simulink model "Simulation_2018"  (R2022b)
settings: Solver=FixedStepAuto  StartTime=0.0  StopTime=Tsim  FixedStep=param.tSample  RelTol=1e-3  EnableMultiTasking=on
StopFcn:
  | run animation
  | run plotSol
values from neighbouring files (symbols this model uses):
  grampc = grampc_update_struct_grampc(grampc,user)    [initData.m]
  param = load_parameter(param)    [script_Simulation.m]
undefined symbols (not defined in the file or in its folder): cost
settings Model: Creator=kaepernick  LastModifiedBy=Khaled
settings SolverCC: AlgebraicLoopSolver=TrustRegion
settings DataIOCC: LimitDataPoints=on  SaveFormat=Array  ReturnWorkspaceOutputs=off
settings OptimizationCC: ExpressionDepthLimit=2147483647  LifeSpan=inf
settings DebuggingCC: UnderspecifiedInitializationDetection=Classic  MergeDetectMultiDrivingBlocksExec=none  SolverPrmCheckMsg=warning  UnconnectedInputMsg=warning  UnconnectedOutputMsg=warning  UnconnectedLineMsg=warning  StateNameClashWarn=warning  SFUnexpectedBacktrackingDiag=warning  SFNoUnconditionalDefaultTransitionDiag=warning  SFExecutionAtInitializationDiag=none  SFMachineParentedDataDiag=warning  ArithmeticOperatorsInVariantConditions=warning
settings HardwareCC: ProdBitPerPointer=32  ProdBitPerSizeT=32  ProdBitPerPtrDiffT=32  ProdLargestAtomicFloat=None  ProdIntDivRoundTo=Undefined  ProdEndianess=Unspecified  ProdWordSize=32  ProdHWDeviceType=32-bit Generic
settings ModelReferenceCC: EnableRefExpFcnMdlSchedulingChecks=on  PropagateSignalLabelsOutOfModel=off
settings SFSimCC: SimUseLocalCustomCode=off  CustomCodeUndefinedFunction=UseInterfaceOnly
settings RTWCC: RTWUseLocalCustomCode=off
settings CodeAppCC: StateflowObjectComments=on
settings GRTTargetCC: TargetLangStandard=C89/C90 (ANSI)
settings ConfigComp: CovMetricSettings=dw  CovSaveCumulativeToWorkspaceVar=on  CovSaveSingleToWorkspaceVar=on  CovExternalEMLEnable=off

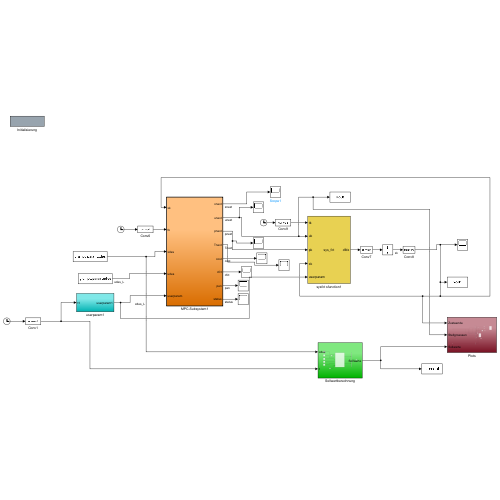
[thumbnail: Simulink's stored preview of the top-level diagram]
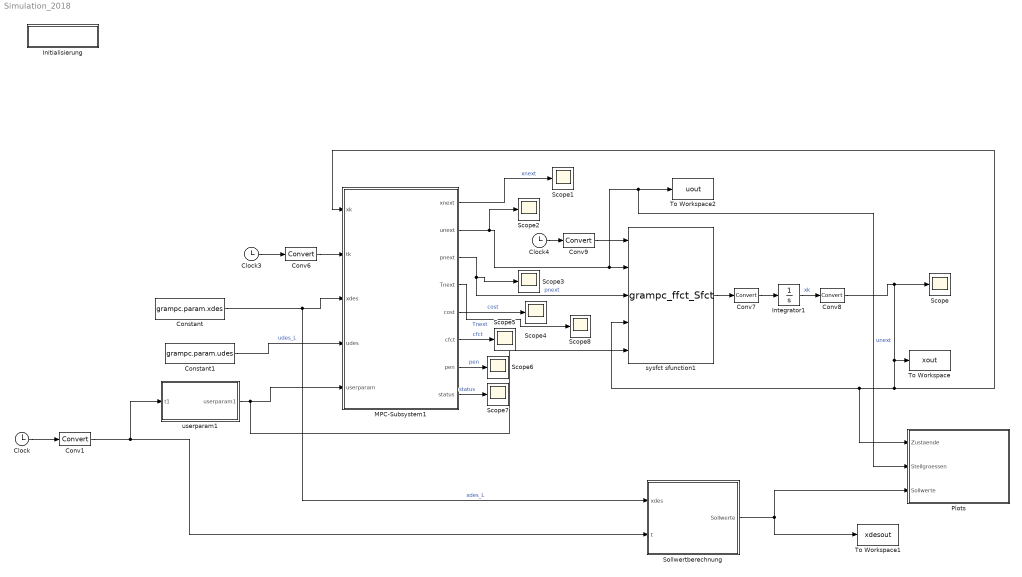
== system Simulation_2018 ==
  Clock : Clock
  Clock3 : Clock
  Clock4 : Clock
  Constant : Constant  Value=grampc.param.xdes
  Constant1 : Constant  Value=grampc.param.udes
  Conv{1,6..9} (5 alike) : DataTypeConversion  SaturateOnIntegerOverflow=off  RndMeth=Floor
  Initialisierung : Subsystem
      settings: OpenFcn=run script_Simulation
  Integrator1 : Integrator  InitialCondition=double(grampc.param.x0)
  MPC-Subsystem1 : Subsystem  TreatAsAtomicUnit=on  SystemSampleTime=double(grampc.param.dt)
  Plots : Subsystem
  Scope{,1..8} (9 alike) : Scope
  Sollwertberechnung : Subsystem
  To Workspace : ToWorkspace  VariableName=xout  SaveFormat=Timeseries  SampleTime=-1
  To Workspace1 : ToWorkspace  VariableName=xdesout  SaveFormat=Timeseries  SampleTime=-1
  To Workspace2 : ToWorkspace  VariableName=uout  SaveFormat=Timeseries  SampleTime=-1
  sysfct sfunction1 : S-Function  FunctionName=grampc_ffct_Sfct  SFunctionDeploymentMode=off  EnableBusSupport=off
      mask Display:
      | port_label('input',1,'tk')
      | port_label('input',2,'uk')
      | port_label('input',3,'pk')
      | port_label('input',4,'xk')
      | port_label('input',5,'userparam')
      | 
      | port_label('output',1,'dfdx')
      | 
      | 
      | disp('sys_fct')
  userparam1 : Subsystem
  wires:
  Sollwertberechnung/1(Sollwerte) -> To Workspace1/1, Plots/3(Sollwerte)
  Clock/1 -> Conv1/1
  Conv1/1 -> userparam1/1(t1), Sollwertberechnung/2(t)
  Constant/1 -> MPC-Subsystem1/3(xdes), Sollwertberechnung/1(xdes)  "xdes_L"
  Conv6/1 -> MPC-Subsystem1/2(tk)
  Clock3/1 -> Conv6/1
  Constant1/1 -> MPC-Subsystem1/4(udes)  "udes_L"
  userparam1/1(userparam1) -> sysfct sfunction1/5, MPC-Subsystem1/5(userparam)
  sysfct sfunction1/1 -> Conv7/1
  Integrator1/1 -> Conv8/1  "xk"
  Conv7/1 -> Integrator1/1
  Clock4/1 -> Conv9/1
  Conv9/1 -> sysfct sfunction1/1
  MPC-Subsystem1/2(unext) -> Scope2/1, Plots/2(Stellgroessen), To Workspace2/1, sysfct sfunction1/2  "unext"
  MPC-Subsystem1/3(pnext) -> Scope3/1, sysfct sfunction1/3  "pnext"
  Conv8/1 -> To Workspace/1, Plots/1(Zustaende), sysfct sfunction1/4, MPC-Subsystem1/1(xk), Scope/1
  MPC-Subsystem1/1(xnext) -> Scope1/1  "xnext"
  MPC-Subsystem1/5(cost) -> Scope4/1  "cost"
  MPC-Subsystem1/6(cfct) -> Scope5/1  "cfct"
  MPC-Subsystem1/7(pen) -> Scope6/1  "pen"
  MPC-Subsystem1/8(status) -> Scope7/1  "status"
  MPC-Subsystem1/4(Tnext) -> Scope8/1  "Tnext"

== system Simulation_2018/Initialisierung ==

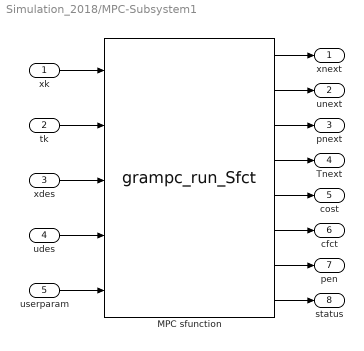
== system Simulation_2018/MPC-Subsystem1 ==
  xk : Inport
  tk : Inport  Port=2
  xdes : Inport  Port=3
  udes : Inport  Port=4
  userparam : Inport  Port=5
  MPC sfunction : S-Function  FunctionName=grampc_run_Sfct  Parameters=grampc_sdata.intoptidx grampc_sdata.intopt grampc_sdata.numoptidx grampc_sdata.numopt grampc_sdata.numparamidx grampc_sdata.numparam  SFunctionDeploymentMode=off  EnableBusSupport=off
      mask Display:
      | port_label('input',1,'x0')
      | port_label('input',2,'t0')
      | port_label('input',3,'xdes')
      | port_label('input',4,'udes')
      | port_label('input',5,'userparam')
      | 
      | port_label('output',1,'xnext')
      | port_label('output',2,'unext')
      | port_label('output',3,'pnext')
      | port_label('output',4,'Tnext')
      | port_label('output',5,'cost')
      | port_label('output',6,'||cfct||')
      | port_label('output',7,'||pen||')
      | port_label('output',8,'status')
      | 
      | disp('GRAMPC')
  xnext : Outport  VectorParamsAs1DForOutWhenUnconnected=off
  unext : Outport  Port=2  VectorParamsAs1DForOutWhenUnconnected=off
  pnext : Outport  Port=3  VectorParamsAs1DForOutWhenUnconnected=off
  Tnext : Outport  Port=4  VectorParamsAs1DForOutWhenUnconnected=off
  cost : Outport  Port=5  VectorParamsAs1DForOutWhenUnconnected=off
  cfct : Outport  Port=6  VectorParamsAs1DForOutWhenUnconnected=off
  pen : Outport  Port=7  VectorParamsAs1DForOutWhenUnconnected=off
  status : Outport  Port=8  VectorParamsAs1DForOutWhenUnconnected=off
  wires:
  xk/1 -> MPC sfunction/1
  MPC sfunction/1 -> xnext/1
  MPC sfunction/8 -> status/1
  MPC sfunction/7 -> pen/1
  xdes/1 -> MPC sfunction/3
  MPC sfunction/6 -> cfct/1
  udes/1 -> MPC sfunction/4
  MPC sfunction/5 -> cost/1
  MPC sfunction/3 -> pnext/1
  MPC sfunction/4 -> Tnext/1
  MPC sfunction/2 -> unext/1
  tk/1 -> MPC sfunction/2
  userparam/1 -> MPC sfunction/5

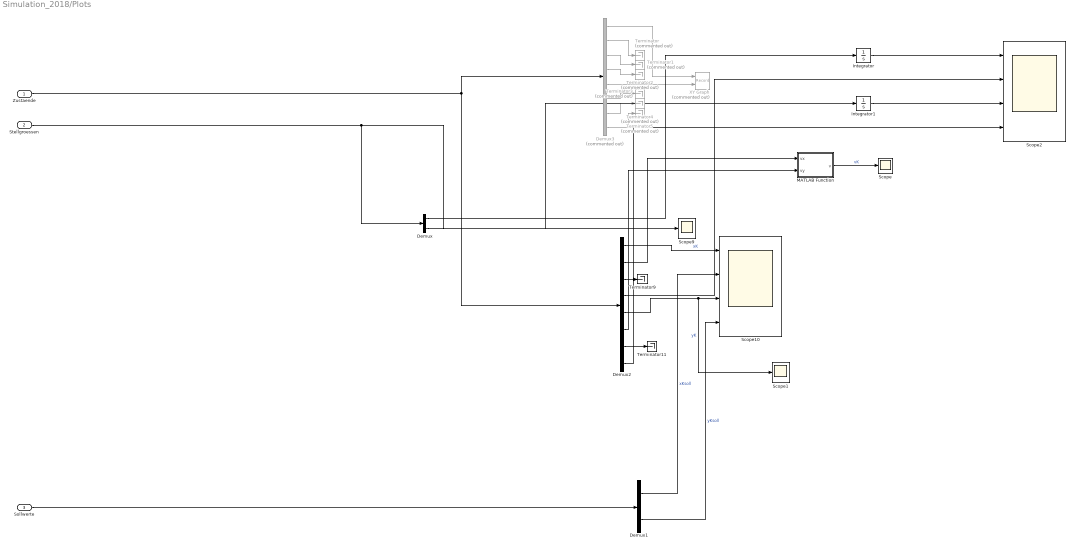
== system Simulation_2018/Plots ==
  Zustaende : Inport
  Stellgroessen : Inport  Port=2
  Sollwerte : Inport  Port=3
  Demux : Demux  Outputs=2
  Demux1 : Demux  Outputs=2
  Demux2 : Demux  Outputs=8
  Demux3 : Demux  Commented=on  Outputs=8
  Integrator : Integrator
  Integrator1 : Integrator
  MATLAB Function : MATLAB Function  TreatAsAtomicUnit=on
  Scope : Scope
  Scope1 : Scope
  Scope10 : Scope  NumInputPorts=4
  Scope2 : Scope  NumInputPorts=4
  Scope9 : Scope
  Terminator{,1..5} (6 alike) : Terminator  Commented=on
  Terminator11 : Terminator
  Terminator9 : Terminator
  XY Graph : Record  Commented=on  FileSettingsInternal="{\"entries\":[{\"content\":{\"excelSettings\":{\"content\":{},\"type\":\"Streamout.ExcelSettings\"}},\"type\":\"Streamout.FileSettingStorage\",\"uuid\":\"823fc073-f533-4fd2-9304-fd0138ba539a\"}],\"packageUris\":[\"http://schema.mathworks.com/mf0/streamout_blocks/R2020a\"],\"version\":\"1.0\"}"  Layout=[1 1]  SignalsInternal="{\"entries\":[{\"content\":{\"signals\":[{\"content\":{\"blockPath\":[\"Simulation_2018/Plots/XY Graph\"],\"channel\":[],\"dimensions\":[1],\"domain\":\"Simulation_2018/Plots/XY Graph\",\"lineColor\":\"#a2142f\",\"plots\":[1],\"port\":1,\"sid\":[],\"signalID\":122,\"signalName\":\"XY Graph:1\"},\"type\":\"RecordBlkView.Signal\",\"uuid\":\"b63b5092-08b6-42c8-9337-63953eef31e7\"},{\"content\":{\"blockPath\":[\"Simulation_2018/Plots/XY Graph\"],\"channel\":[],\"dimensions\":[1],\"domain\":\"Simulation_2018/Plots/XY Graph\",\"lineColor\":\"#139fff\",\"plots\":[1],\"port\":2,\"sid\":[],\"signalID\":125,\"signalName\":\"XY Graph:2\"},\"type\":\"RecordBlkView.Signal\",\"uuid\":\"3b01fe3b-a78f-42cf-b061-e2f77cf29949\"}]},\"type\":\"RecordBlkView.InputSignals\",\"uuid\":\"8815cdad-7d21-4a19-9d66-34a392429214\"}],\"packageUris\":[\"http://schema.mathworks.com/mf0/streamout_blocks/R2020a\"],\"version\":\"1.0\"}"  VisualizationBindings="{\"xyplotplugin\":{\"info\":[{\"series\":[{\"bindingParametersList\":[{\"parameter\":\"X-Axis\",\"signalID\":122,\"signalName\":\"XY Graph:1\"},{\"parameter\":\"Y-Axis\",\"signalID\":125,\"signalName\":\"XY Graph:2\"}],\"seriesID\":53896}],\"subplotID\":1}]}}"  CompatibilityTag=XY  st=-1
  wires:
  Demux2/6 -> MATLAB Function/2(vy)
  Demux1/2 -> Scope10/4  "yKsoll"
  Demux2/5 -> Scope1/1, Scope10/3  "yK"
  Demux2/2 -> MATLAB Function/1(vx)
  Demux3/1 -> XY Graph/1
  Demux2/1 -> Scope10/1  "xK"
  Demux3/5 -> XY Graph/2
  Demux1/1 -> Scope10/2  "xKsoll"
  Zustaende/1 -> Demux2/1, Demux3/1
  Sollwerte/1 -> Demux1/1
  Stellgroessen/1 -> Demux/1, Scope9/1
  Demux3/2 -> Terminator/1
  Demux3/3 -> Terminator1/1
  Demux3/4 -> Terminator2/1
  Demux3/6 -> Terminator3/1
  Demux3/7 -> Terminator4/1
  Demux3/8 -> Terminator5/1
  Demux2/3 -> Terminator9/1
  Demux2/4 -> Scope2/2
  Demux2/7 -> Terminator11/1
  Demux2/8 -> Scope2/4
  Demux/1 -> Integrator/1
  Demux/2 -> Integrator1/1
  Integrator/1 -> Scope2/1
  Integrator1/1 -> Scope2/3
  MATLAB Function/1(v) -> Scope/1  "vK"

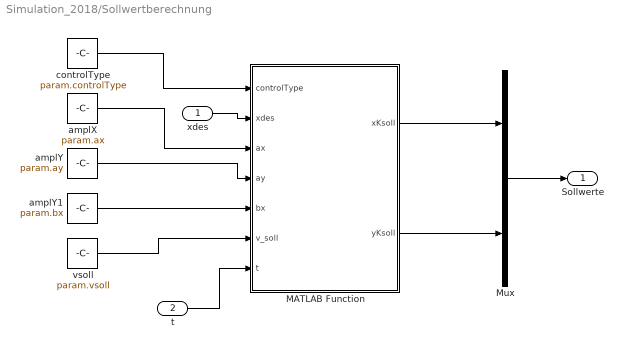
== system Simulation_2018/Sollwertberechnung ==
  xdes : Inport
  t : Inport  Port=2
  MATLAB Function : MATLAB Function  TreatAsAtomicUnit=on
  Mux : Mux  Inputs=2
  amplX : Constant  Value=param.ax
  amplY : Constant  Value=param.ay
  amplY1 : Constant  Value=param.bx
  controlType : Constant  Value=param.controlType
  vsoll : Constant  Value=param.vsoll
  Sollwerte : Outport  VectorParamsAs1DForOutWhenUnconnected=off
  wires:
  Mux/1 -> Sollwerte/1
  MATLAB Function/1(xKsoll) -> Mux/1
  MATLAB Function/2(yKsoll) -> Mux/2
  controlType/1 -> MATLAB Function/1(controlType)
  amplX/1 -> MATLAB Function/3(ax)
  amplY/1 -> MATLAB Function/4(ay)
  vsoll/1 -> MATLAB Function/6(v_soll)
  xdes/1 -> MATLAB Function/2(xdes)
  t/1 -> MATLAB Function/7(t)
  amplY1/1 -> MATLAB Function/5(bx)

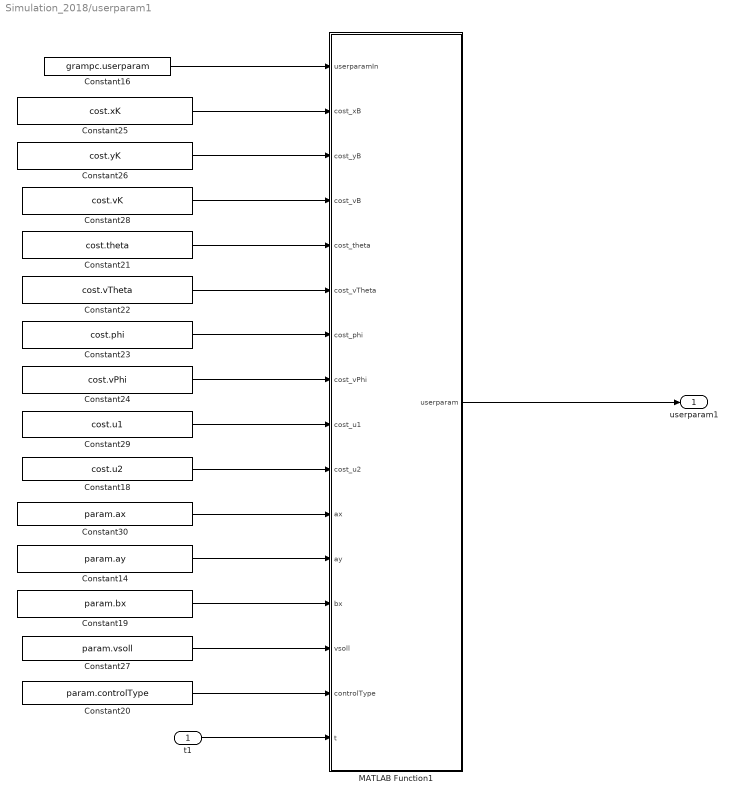
== system Simulation_2018/userparam1 ==
  t1 : Inport
  Constant14 : Constant  Value=param.ay
  Constant16 : Constant  Value=grampc.userparam
  Constant18 : Constant  Value=cost.u2
  Constant19 : Constant  Value=param.bx
  Constant20 : Constant  Value=param.controlType
  Constant21 : Constant  Value=cost.theta
  Constant22 : Constant  Value=cost.vTheta
  Constant23 : Constant  Value=cost.phi
  Constant24 : Constant  Value=cost.vPhi
  Constant25 : Constant  Value=cost.xK
  Constant26 : Constant  Value=cost.yK
  Constant27 : Constant  Value=param.vsoll
  Constant28 : Constant  Value=cost.vK
  Constant29 : Constant  Value=cost.u1
  Constant30 : Constant  Value=param.ax
  MATLAB Function1 : MATLAB Function  TreatAsAtomicUnit=on
  userparam1 : Outport  VectorParamsAs1DForOutWhenUnconnected=off
  wires:
  t1/1 -> MATLAB Function1/16(t)
  Constant25/1 -> MATLAB Function1/2(cost_xB)
  Constant30/1 -> MATLAB Function1/11(ax)
  Constant22/1 -> MATLAB Function1/6(cost_vTheta)
  Constant29/1 -> MATLAB Function1/9(cost_u1)
  Constant16/1 -> MATLAB Function1/1(userparamIn)
  Constant18/1 -> MATLAB Function1/10(cost_u2)
  Constant26/1 -> MATLAB Function1/3(cost_yB)
  Constant14/1 -> MATLAB Function1/12(ay)
  Constant20/1 -> MATLAB Function1/15(controlType)
  Constant19/1 -> MATLAB Function1/13(bx)
  Constant23/1 -> MATLAB Function1/7(cost_phi)
  MATLAB Function1/1(userparam) -> userparam1/1
  Constant27/1 -> MATLAB Function1/14(vsoll)
  Constant28/1 -> MATLAB Function1/4(cost_vB)
  Constant21/1 -> MATLAB Function1/5(cost_theta)
  Constant24/1 -> MATLAB Function1/8(cost_vPhi)

== matlab function Simulation_2018/Plots/MATLAB Function ==
  data: vx input; v output; vy input
function v = fcn(vx, vy)

v = sqrt(vx*vx+vy*vy);

== matlab function Simulation_2018/Sollwertberechnung/MATLAB Function ==
  data: controlType input; xdes input; ax input; xKsoll output; ay input; bx input; v_soll input; yKsoll output; t input
function [xKsoll,yKsoll] = fcn(controlType, xdes, ax, ay, bx, v_soll, t)
    
    %TODO
   
    % AP-Wechsel / Setpoint change
    xKsoll = 0;
	yKsoll = 0.15;
    
    % Trajektorienfolgeregelung / Trajectory tracking
    if controlType == 1
        xKsoll = ax * sin(bx * v_soll *t);
        yKsoll = ay * cos(v_soll *t);
    end
    
end

== matlab function Simulation_2018/userparam1/MATLAB Function1 ==
  data: userparamIn input; userparam output; cost_xB input; cost_yB input; cost_vB input; cost_theta input; cost_vTheta input; cost_phi input; cost_vPhi input; cost_u1 input; cost_u2 input; ax input; ay input; bx input; vsoll input; controlType input; t input
function userparam   = fcn(userparamIn, cost_xB, cost_yB, cost_vB, ... 
    cost_theta, cost_vTheta, cost_phi, cost_vPhi, ...
    cost_u1, cost_u2, ...
    ax, ay, bx, vsoll, ...
    controlType, t)

userparam = userparamIn;

userparam(1) = cost_xB;
userparam(2) = cost_yB;
userparam(3) = cost_vB;

userparam(4) = cost_theta;
userparam(5) = cost_vTheta;
userparam(6) = cost_phi;
userparam(7) = cost_vPhi;

userparam(8) = cost_u1;
userparam(9) = cost_u2;

userparam(10) = ax;
userparam(11) = ay;
userparam(12) = bx;
userparam(13) = vsoll;

userparam(14) = controlType;

userparam(15) = t;
